simulink model "coupled_msd_4"  (R2022a)
settings: Solver=VariableStepAuto  StartTime=0.0  StopTime=T  RelTol=1e-3
values from neighbouring files (symbols this model uses):
  sys_par = data_config.system    [init_klmn.m]    (also in static_ozf.m)
  x0 = data_config.simulator.initial_state    [init_klmn.m]    (also in static_ozf.m)
settings Model: Creator=jack  LastModifiedBy=jack

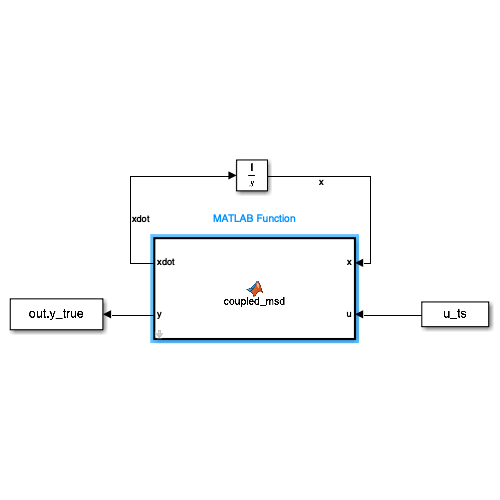
[thumbnail: Simulink's stored preview of the top-level diagram]
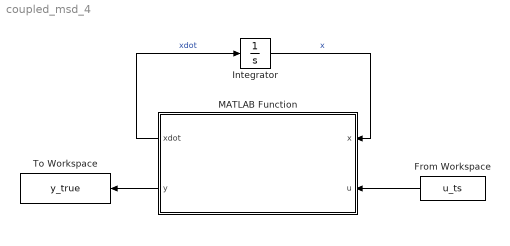
== system coupled_msd_4 ==
  From Workspace : FromWorkspace  VariableName=u_ts
  Integrator : Integrator  InitialCondition=x0
  MATLAB Function : MATLAB Function  TreatAsAtomicUnit=on  mask{C_out=sys_par.C, m=sys_par.m, c=sys_par.c, k=sys_par.k}
  To Workspace : ToWorkspace  VariableName=y_true  SaveFormat=Timeseries  SampleTime=-1
  wires:
  MATLAB Function/1(xdot) -> Integrator/1  "xdot"
  Integrator/1 -> MATLAB Function/1(x)  "x"
  From Workspace/1 -> MATLAB Function/2(u)
  MATLAB Function/2(y) -> To Workspace/1

== matlab function coupled_msd_4/MATLAB Function ==
  data: x input; xdot output; u input; y output; m parameter; k parameter; c parameter; C_out parameter
function [xdot,y] = coupled_msd(x,u, m, k, c, C_out)

y = C_out*x;
xdot = [
    x(2);
    1/m(1)*(u+  k(1)*Gamma(     -x(1))+     k(2)*Gamma(x(3)-x(1)) + c(1)*(      -x(2))+     c(2)*(x(4)- x(2)));
    x(4);
    1/m(2)*(    k(2)*Gamma(x(1) -x(3))+     k(3)*Gamma(x(5)-x(3)) + c(2)*(x(2)  -x(4))+     c(3)*(x(6)- x(4)));
    x(6);
    1/m(3)*(    k(3)*Gamma(x(3) -x(5))+     k(4)*Gamma(x(7)-x(5)) + c(3)*(x(4)  -x(6))+     c(4)*(x(8)- x(6)));
    x(8);
    1/m(4)*(    k(4)*Gamma(x(5) -x(7))+                             c(4)*(x(6)  -x(8)))
];
